simulink model "finalsim"  (R2024a)
settings: Solver=FixedStepAuto  StartTime=0.0  StopTime=sat.sim_time  FixedStep=0.1  RelTol=1e-3
undefined symbols (not defined in the file or in its folder): compact, sat, WMM2020
libraries: aerolibutil x10, matrix_library x2, aerolibgravity2 x1
settings Model: Creator=aryam  LastModifiedBy=ashis
settings ModelReferenceCC: ModelReferenceNumInstancesAllowed=Single
settings RTWCC: GPUComputeCapability=3.5

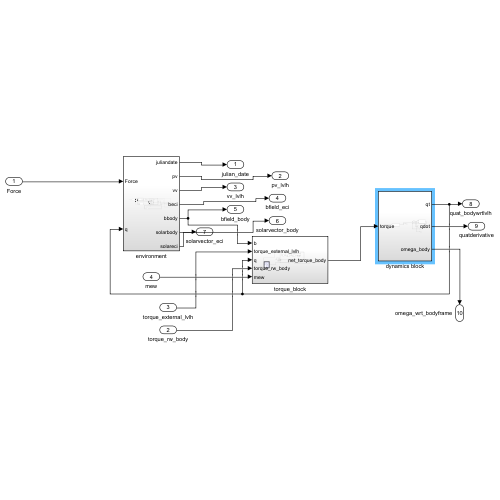
[thumbnail: Simulink's stored preview of the top-level diagram]
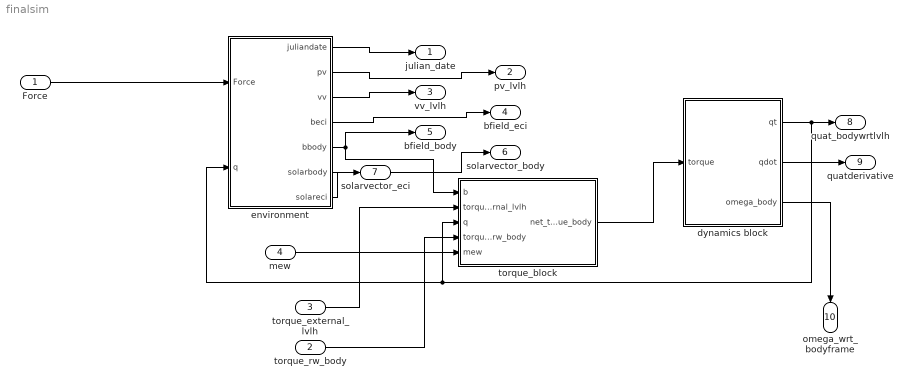
== system finalsim ==
  Force : Inport  PortDimensions=3
  torque_rw_body : Inport  Port=2  PortDimensions=3
  torque_external_lvlh : Inport  Port=3  PortDimensions=3
  mew : Inport  Port=4  PortDimensions=3
  dynamics block : Subsystem
  environment : Subsystem
  torque_block : Subsystem
  julian_date : Outport
  pv_lvlh : Outport  Port=2
  vv_lvlh : Outport  Port=3
  bfield_eci : Outport  Port=4
  bfield_body : Outport  Port=5
  solarvector_body : Outport  Port=6
  solarvector_eci : Outport  Port=7
  quat_bodywrtlvlh : Outport  Port=8
  quatderivative : Outport  Port=9
  omega_wrt_bodyframe : Outport  Port=10
  wires:
  dynamics block/1(qt) -> quat_bodywrtlvlh/1, torque_block/3(q), environment/2(q)
  Force/1 -> environment/1(Force)
  environment/5(bbody) -> bfield_body/1, torque_block/1(b)
  torque_external_lvlh/1 -> torque_block/2(torque_external_lvlh)
  torque_rw_body/1 -> torque_block/4(torque_rw_body)
  torque_block/1(net_torque_body) -> dynamics block/1(torque)
  environment/1(juliandate) -> julian_date/1
  environment/2(pv) -> pv_lvlh/1
  environment/3(vv) -> vv_lvlh/1
  environment/4(beci) -> bfield_eci/1
  environment/6(solarbody) -> solarvector_body/1
  environment/7(solareci) -> solarvector_eci/1
  mew/1 -> torque_block/5(mew)
  dynamics block/2(qdot) -> quatderivative/1
  dynamics block/3(omega_body) -> omega_wrt_bodyframe/1

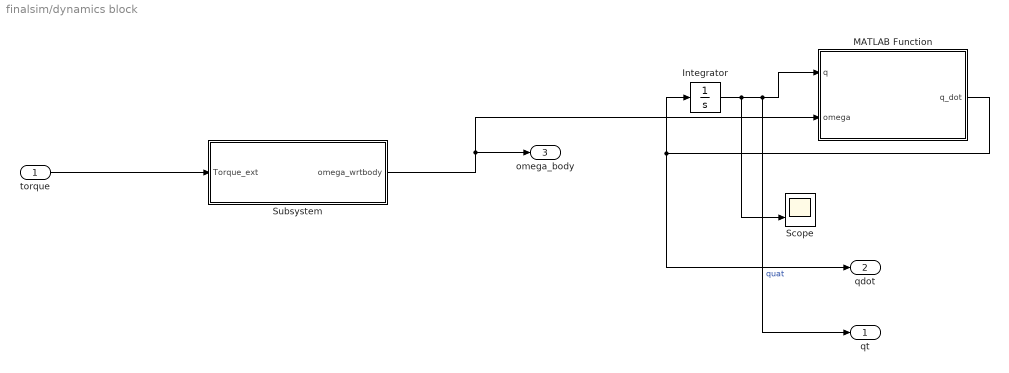
== system finalsim/dynamics block ==
  torque : Inport
  Integrator : Integrator  InitialCondition=compact(sat.initialorientation)
  MATLAB Function : MATLAB Function  TreatAsAtomicUnit=on
  Scope : Scope  NumInputPorts=2
  Subsystem : Subsystem
  qt : Outport
  qdot : Outport  Port=2
  omega_body : Outport  Port=3
  wires:
  torque/1 -> Subsystem/1(Torque_ext)
  Subsystem/1(omega_wrtbody) -> MATLAB Function/2(omega), omega_body/1
  Integrator/1 -> qt/1, MATLAB Function/1(q), Scope/2  "quat"
  MATLAB Function/1(q_dot) -> Integrator/1, qdot/1

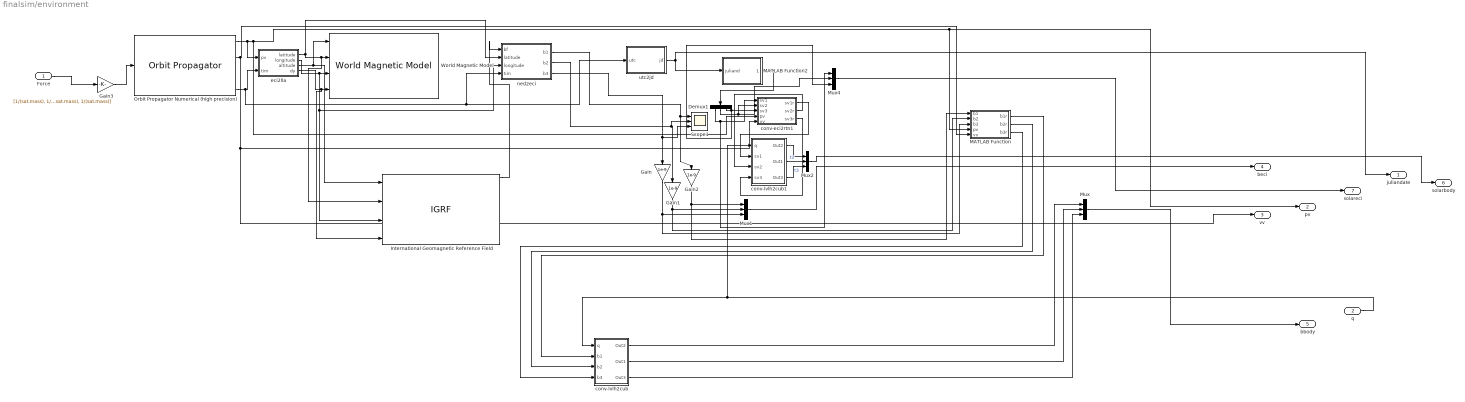
== system finalsim/environment ==
  Force : Inport
  q : Inport  Port=2
  Demux1 : Demux  Outputs=3
  Gain : Gain  Gain=1e-9
  Gain1 : Gain  Gain=1e-9
  Gain2 : Gain  Gain=1e-9
  Gain3 : Gain  Gain=[1/(sat.mass), 1/(sat.mass), 1/(sat.mass)]
  International Geomagnetic Reference Field : IGRF  month=January  day=1  year=2020
      settings: AttributesFormatString=%<generation>
  MATLAB Function : MATLAB Function  TreatAsAtomicUnit=on
  MATLAB Function2 : MATLAB Function  TreatAsAtomicUnit=on
  Mux{,1..2,4} (4 alike) : Mux  Inputs=3
  Orbit Propagator Numerical (high precision) : OrbitPropagator  propagator=Numerical (high precision)  accelIn=on  startDate=sat.starttime  mass=sat.mass  semiMajorAxis=sat.orb.sma  eccentricity=sat.orb.ecc  inclination=sat.orb.inc  raan=sat.orb.raan  argPeriapsis=sat.orb.peri  trueAnomaly=sat.orb.theta  inertialPosition=[3649700.0 3308200.0 -4676600.0]  inertialVelocity=[-2750.8 6666.4 2573.4]  fixedPosition=[-4142689.0 -2676864.7 -4669861.6]  fixedVelocity=[1452.7 -6720.7 2568.1]  customR=3396200  customMu=4.305e13  customJ2=1.0826269e-03  customOmega=4.06125949e-3  outputTransform=on  useDrag=on  F107ExtrapMethod=Least squares fit  MagneticIndexExtrapMethod=IGRF  dragCoeff=sat.dragco  dragArea=sat.dragarea  ephemerisModel=DE432t  timeFormat=Gregorian
  Scope1 : Scope  NumInputPorts=3
  World Magnetic Model : aerolibgravity2/World Magnetic Model  model=WMM2020 (2020-2025)  customFile='WMM2020.COF'  units=Metric (MKS)  time_in=on  month=January  day=1  year=2020  action=Error  h_out=off  dec_out=off  inc_out=off  ti_out=off
  conv-eci2rtn1 : MATLAB Function  TreatAsAtomicUnit=on
  conv-lvlh2cub : Subsystem
  conv-lvlh2cub1 : Subsystem
  eci2lla : MATLAB Function  TreatAsAtomicUnit=on
  ned2eci : MATLAB Function  TreatAsAtomicUnit=on
  utc2jd : MATLAB Function  TreatAsAtomicUnit=on
  juliandate : Outport
  pv : Outport  Port=2
  vv : Outport  Port=3
  beci : Outport  Port=4
  bbody : Outport  Port=5
  solarbody : Outport  Port=6
  solareci : Outport  Port=7
  wires:
  Mux/1 -> bbody/1
  Orbit Propagator Numerical (high precision)/2 -> vv/1, conv-eci2rtn1/5(vv), MATLAB Function/5(vv)
  Mux1/1 -> beci/1
  utc2jd/1(jd) -> juliandate/1, MATLAB Function2/1(juliand)
  Mux2/1 -> solarbody/1
  Orbit Propagator Numerical (high precision)/1 -> pv/1, MATLAB Function/4(pv), conv-eci2rtn1/4(pv), eci2lla/1(pv)
  Mux4/1 -> solareci/1
  MATLAB Function/1(b1r) -> conv-lvlh2cub/2(b1)
  MATLAB Function/2(b2r) -> conv-lvlh2cub/3(b2)
  MATLAB Function/3(b3r) -> conv-lvlh2cub/4(b3)
  conv-lvlh2cub/3(Out3) -> Mux/3
  conv-lvlh2cub/2(Out1) -> Mux/2
  Force/1 -> Gain3/1
  Demux1/3 -> Mux4/3, conv-eci2rtn1/3(sv3)
  Demux1/1 -> Mux4/1, conv-eci2rtn1/1(sv1)
  ned2eci/1(b1) -> Scope1/1, Gain2/1
  eci2lla/1(latitude) -> International Geomagnetic Reference Field/2, World Magnetic Model/2, ned2eci/2(latitude)
  Orbit Propagator Numerical (high precision)/4 -> utc2jd/1(utc), ned2eci/4(tim), eci2lla/2(tim)
  ned2eci/3(b3) -> Gain/1, Scope1/3
  eci2lla/3(altitude) -> International Geomagnetic Reference Field/1, World Magnetic Model/1
  Gain2/1 -> MATLAB Function/1(b1), Mux1/1
  conv-eci2rtn1/3(sv3r) -> conv-lvlh2cub1/4(sv3)
  q/1 -> conv-lvlh2cub1/1(q), conv-lvlh2cub/1(q)
  Gain1/1 -> MATLAB Function/2(b2), Mux1/2
  conv-lvlh2cub1/3(Out3) -> Mux2/3  "t3"
  conv-lvlh2cub1/1(Out2) -> Mux2/1
  Gain3/1 -> Orbit Propagator Numerical (high precision)/1
  eci2lla/4(dy) -> International Geomagnetic Reference Field/4, World Magnetic Model/4
  conv-eci2rtn1/1(sv1r) -> conv-lvlh2cub1/2(sv1)
  Gain/1 -> MATLAB Function/3(b3), Mux1/3
  conv-lvlh2cub1/2(Out1) -> Mux2/2  "t2"
  ned2eci/2(b2) -> Gain1/1, Scope1/2
  MATLAB Function2/1(solarvector) -> Demux1/1
  conv-eci2rtn1/2(sv2r) -> conv-lvlh2cub1/3(sv2)
  eci2lla/2(longitude) -> ned2eci/3(longitude), International Geomagnetic Reference Field/3, World Magnetic Model/3
  Demux1/2 -> Mux4/2, conv-eci2rtn1/2(sv2)
  conv-lvlh2cub/1(Out2) -> Mux/1
  International Geomagnetic Reference Field/1 -> ned2eci/1(bf)

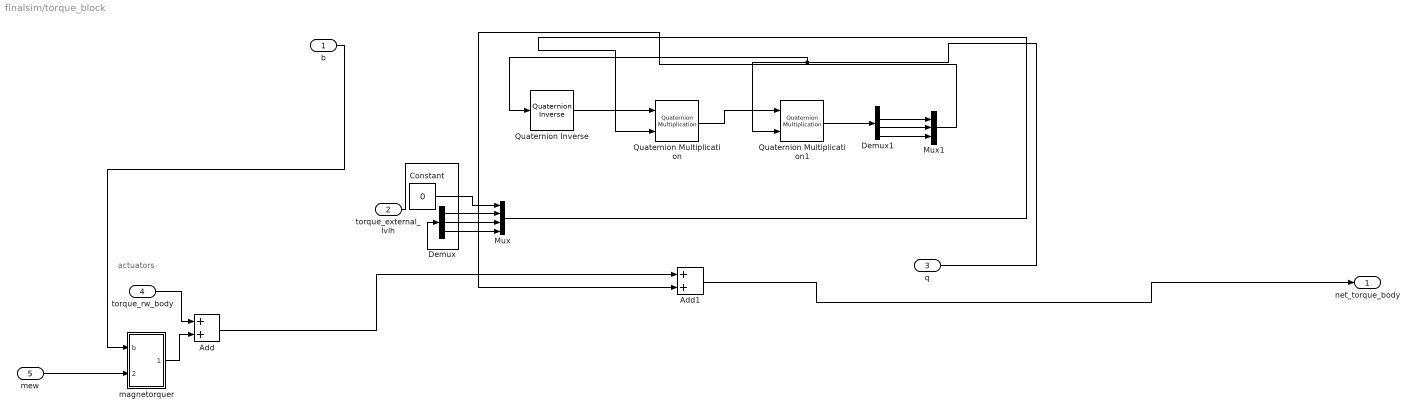
== system finalsim/torque_block ==
  note: actuators
  b : Inport
  torque_external_lvlh : Inport  Port=2
  q : Inport  Port=3
  torque_rw_body : Inport  Port=4
  mew : Inport  Port=5
  Add : Sum
  Add1 : Sum
  Constant : Constant  Value=0
  Demux : Demux  Outputs=3
  Demux1 : Demux
  Mux : Mux
  Mux1 : Mux  Inputs=3
  Quaternion Inverse : aerolibutil/Quaternion Inverse
  Quaternion Multiplication : aerolibutil/Quaternion Multiplication
  Quaternion Multiplication1 : aerolibutil/Quaternion Multiplication
  magnetorquer : Subsystem
  net_torque_body : Outport
  wires:
  Demux1/4 -> Mux1/3
  Quaternion Multiplication/1 -> Quaternion Multiplication1/1
  Demux/3 -> Mux/4
  Quaternion Multiplication1/1 -> Demux1/1
  magnetorquer/1(torque_body) -> Add/2
  torque_external_lvlh/1 -> Demux/1
  Demux1/3 -> Mux1/2
  Demux1/2 -> Mux1/1
  Demux/1 -> Mux/2
  Add/1 -> Add1/1
  Quaternion Inverse/1 -> Quaternion Multiplication/1
  Constant/1 -> Mux/1
  Demux/2 -> Mux/3
  torque_rw_body/1 -> Add/1
  Add1/1 -> net_torque_body/1
  b/1 -> magnetorquer/1(b)
  Mux1/1 -> Add1/2
  q/1 -> Quaternion Multiplication1/2, Quaternion Inverse/1
  Mux/1 -> Quaternion Multiplication/2
  mew/1 -> magnetorquer/2(mew)

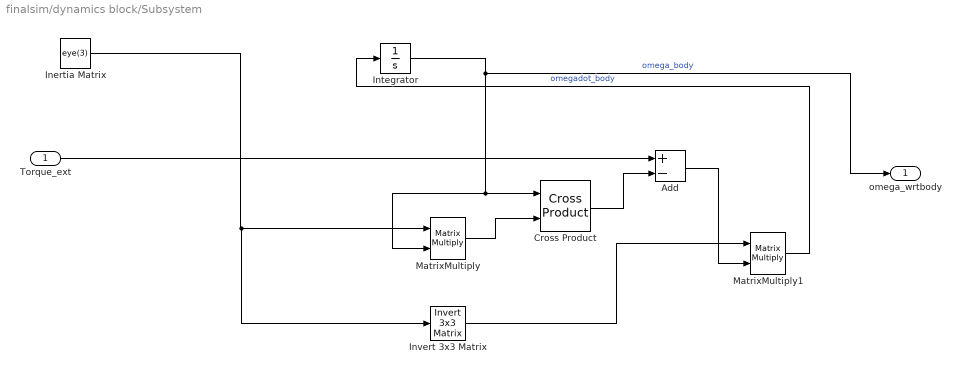
== system finalsim/dynamics block/Subsystem ==
  Torque_ext : Inport  PortDimensions=3
  Add : Sum  Inputs=+-
  Cross Product : matrix_library/Cross Product
  Inertia Matrix : Constant  Value=eye(3)
  Integrator : Integrator  InitialCondition=[0, 0, 0]
  Invert 3x3 Matrix : aerolibutil/Invert  3x3 Matrix
  MatrixMultiply : Product  Multiplication=Matrix(*)
  MatrixMultiply1 : Product  Multiplication=Matrix(*)
  omega_wrtbody : Outport
  wires:
  Add/1 -> MatrixMultiply1/2
  Inertia Matrix/1 -> Invert 3x3 Matrix/1, MatrixMultiply/1
  Integrator/1 -> omega_wrtbody/1, Cross Product/1, MatrixMultiply/2  "omega_body"
  MatrixMultiply1/1 -> Integrator/1  "omegadot_body"
  MatrixMultiply/1 -> Cross Product/2
  Invert 3x3 Matrix/1 -> MatrixMultiply1/1
  Cross Product/1 -> Add/2
  Torque_ext/1 -> Add/1

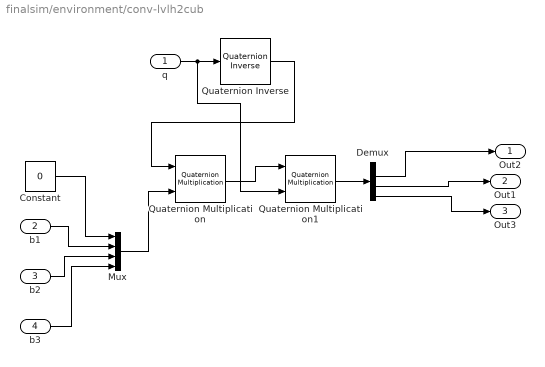
== system finalsim/environment/conv-lvlh2cub ==
  q : Inport
  b1 : Inport  Port=2
  b2 : Inport  Port=3
  b3 : Inport  Port=4
  Constant : Constant  Value=0
  Demux : Demux
  Mux : Mux
  Quaternion Inverse : aerolibutil/Quaternion Inverse
  Quaternion Multiplication : aerolibutil/Quaternion Multiplication
  Quaternion Multiplication1 : aerolibutil/Quaternion Multiplication
  Out2 : Outport
  Out1 : Outport  Port=2
  Out3 : Outport  Port=3
  wires:
  Quaternion Multiplication/1 -> Quaternion Multiplication1/1
  Constant/1 -> Mux/1
  Mux/1 -> Quaternion Multiplication/2
  Demux/4 -> Out3/1
  q/1 -> Quaternion Multiplication1/2, Quaternion Inverse/1
  Quaternion Multiplication1/1 -> Demux/1
  Demux/3 -> Out1/1
  Demux/2 -> Out2/1
  Quaternion Inverse/1 -> Quaternion Multiplication/1
  b1/1 -> Mux/2
  b2/1 -> Mux/3
  b3/1 -> Mux/4

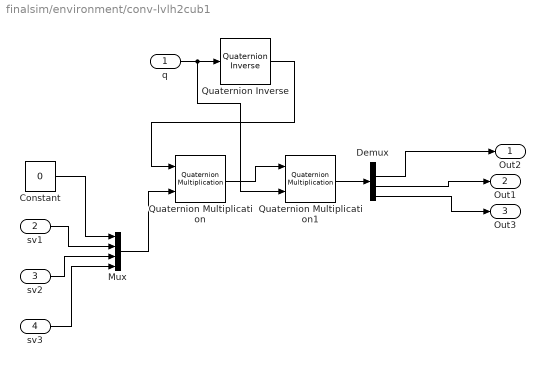
== system finalsim/environment/conv-lvlh2cub1 ==
  q : Inport
  sv1 : Inport  Port=2
  sv2 : Inport  Port=3
  sv3 : Inport  Port=4
  Constant : Constant  Value=0
  Demux : Demux
  Mux : Mux
  Quaternion Inverse : aerolibutil/Quaternion Inverse
  Quaternion Multiplication : aerolibutil/Quaternion Multiplication
  Quaternion Multiplication1 : aerolibutil/Quaternion Multiplication
  Out2 : Outport
  Out1 : Outport  Port=2
  Out3 : Outport  Port=3
  wires:
  Quaternion Multiplication/1 -> Quaternion Multiplication1/1
  Constant/1 -> Mux/1
  Mux/1 -> Quaternion Multiplication/2
  Demux/4 -> Out3/1
  q/1 -> Quaternion Multiplication1/2, Quaternion Inverse/1
  Quaternion Multiplication1/1 -> Demux/1
  Demux/3 -> Out1/1
  Demux/2 -> Out2/1
  Quaternion Inverse/1 -> Quaternion Multiplication/1
  sv1/1 -> Mux/2
  sv2/1 -> Mux/3
  sv3/1 -> Mux/4

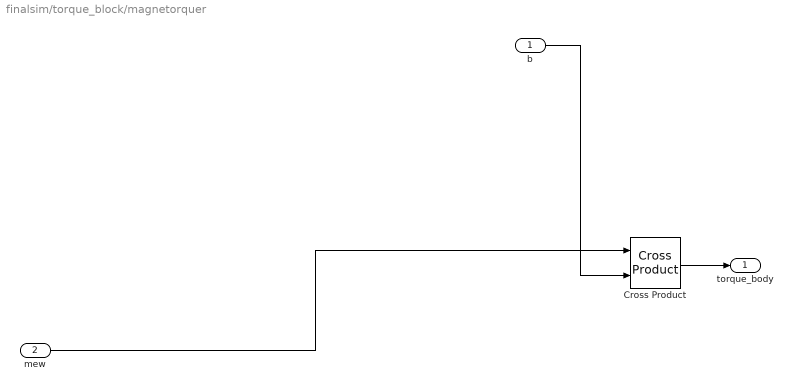
== system finalsim/torque_block/magnetorquer ==
  b : Inport
  mew : Inport  Port=2
  Cross Product : matrix_library/Cross Product
  torque_body : Outport
  wires:
  mew/1 -> Cross Product/1
  Cross Product/1 -> torque_body/1
  b/1 -> Cross Product/2

== matlab function finalsim/environment/ned2eci ==
  data: bf input; b1 output; latitude input; longitude input; tim input; b2 output; b3 output
function [b1, b2, b3] = fcn(bf, latitude, longitude, tim)
    coder.extrinsic("ecef2eci");
    b1=0;
    b2=0;
    b3=0;
    
    bxi=bf(1);
    byi=bf(2);
    bzi=bf(3);
    [bxm, bym, bzm]=(ned2ecefv(bxi, byi, bzi, latitude, longitude));
    bhaha=ecef2eci(tim', [bxm, bym, bzm]);
    b1=bhaha(1);
    b2=bhaha(2);
    b3=bhaha(3);
    
end

== matlab function finalsim/environment/eci2lla ==
  data: pv input; latitude output; tim input; longitude output; altitude output; dy output
function [latitude, longitude, altitude, dy]=  igrf(pv, tim)
    latitude=0;
    longitude=0;
    altitude=0;
    dy=0;
    coder.extrinsic('eci2lla');
    coder.extrinsic('decyear');
    holder=eci2lla(pv', tim');
    latitude=holder(1);
    longitude=holder(2);
    altitude=holder(3);
    dy=decyear(tim');
end

== matlab function finalsim/environment/MATLAB Function ==
  data: b1 input; b1r output; b2 input; b3 input; pv input; vv input; b2r output; b3r output
function [b1r, b2r, b3r] = eci2lvlh(b1, b2, b3, pv, vv)
    thirduv= -pv/norm(pv);
    seconduv=cross(thirduv, vv)/norm(cross(thirduv, vv));
    firstuv=cross(seconduv, thirduv);
     matr=[firstuv, seconduv, thirduv]';
    b=[b1; b2; b3;];
    bnew=matr\b;
    b1r=bnew(1);
    b2r=bnew(2);
    b3r=bnew(3);
end

== matlab function finalsim/environment/utc2jd ==
  data: utc input; jd output
function jd = fcn(utc)
coder.extrinsic('juliandate');
jd=0;
jd = juliandate(utc');

== matlab function finalsim/environment/MATLAB Function2 ==
  data: juliand input; solarvector output
function solarvector = sv_eci(juliand)
% Given Gregorian year(s), day(s), and time(s), calculate Earth-centered
% inertial (ECI) coordinates (in meters) of the vector(s) pointing from
% Earth's center to the center of the Sun.
% Encapsulated by Seth B. Wagenman, from stargazing.net/kepler/sun.html as
% corrected by https://astronomy.stackexchange.com/a/37199/34646 along with
% other minor corrections based on recent revisions to the ecliptic plane.
% Set time(s) relative to the J2000.0 epoch
fractionalDay = juliand - 2451545.0;
% Mean longitude of the Sun

meanLongitudeSunDegrees = 280.4606184 + ...
	((36000.77005361 / 36525) * fractionalDay); %(degrees)
% Mean anomaly of the Sun
meanAnomalySunDegrees = 357.5277233 + ...
	((35999.05034 / 36525) * fractionalDay); %(degrees)
meanAnomalySunRadians = meanAnomalySunDegrees * pi / 180;
% Ecliptic longitude of the Sun
eclipticLongitudeSunDegrees = meanLongitudeSunDegrees + ...
	(1.914666471 * sin(meanAnomalySunRadians)) + ...
	(0.918994643 * sin(2 * meanAnomalySunRadians)); %(degrees)
eclipticLongitudeSunRadians = eclipticLongitudeSunDegrees * pi / 180;
% Obliquity of the ecliptic plane formula mostly derived from:
% https://en.wikipedia.org/wiki/Ecliptic#Obliquity_of_the_ecliptic
epsilonDegrees = ... % Formula deals with time denominated in centuries
	23.43929 - ((46.8093 / 3600) * fractionalDay / 36525);  %(degrees)
epsilonRadians = epsilonDegrees * pi / 180;
% **** Calculations for unit vectors direction to the Sun are in ECI ****
% Now calculate the Earth to Sun unit vector(s) USING RADIANS, NOT DEGREES
unitEarthSunVectorTransposed = [cos(eclipticLongitudeSunRadians).';
    (cos(epsilonRadians) .* sin(eclipticLongitudeSunRadians)).';
    (sin(epsilonRadians) .* sin(eclipticLongitudeSunRadians)).'];
unitEarthSunVector = unitEarthSunVectorTransposed.';
solarvector = -unitEarthSunVector; 
end % End of function

== matlab function finalsim/dynamics block/MATLAB Function ==
  data: q input; q_dot output; omega input
function q_dot = quaternion_derivative(q, omega)
    % q: Quaternion [q0, q1, q2, q3]
    % omega: Angular velocity [omega_x, omega_y, omega_z] in the body frame
    
    % Quaternion components
    q0 = q(1);
    q1 = q(2);
    q2 = q(3);
    q3 = q(4);
    
    % Angular velocity components
    omega_x = omega(1);
    omega_y = omega(2);
    omega_z = omega(3);
    
    % Matrix W(q)
    W = [
        q0, -q1, -q2, -q3;
        q1,  q0, -q3,  q2;
        q2,  q3,  q0, -q1;
        q3, -q2,  q1,  q0;
    ];
    
    % Angular velocity quaternion
    Omega = [0; omega_x; omega_y; omega_z];
    
    % Quaternion derivative
    q_dot_ = 0.5 * W * Omega;
    q_dot=q_dot_';
end

== matlab function finalsim/environment/conv-eci2rtn1 ==
  data: sv1 input; sv1r output; sv2 input; sv3 input; pv input; vv input; sv2r output; sv3r output
function [sv1r, sv2r, sv3r] = eci2lvlh(sv1, sv2, sv3, pv, vv)
    thirduv= -pv/norm(pv);
    seconduv=cross(thirduv, vv)/norm(cross(thirduv, vv));
    firstuv=cross(seconduv, thirduv);
    matr=[firstuv, seconduv, thirduv]';
    b=[sv1; sv2; sv3;];
    bnew=matr\b;
    sv1r=bnew(1);
    sv2r=bnew(2);
    sv3r=bnew(3);
end
